simulink model "Torque_controller"  (R2023b)
settings: Solver=VariableStepAuto  StartTime=0.0  StopTime=50  RelTol=1e-3
values from neighbouring files (symbols this model uses):
  b = 0.016    [torque.m]
  Im = 0.059    [torque.m]
  k = kt    (= 1.45433391507)    [torque.m]
  L = 0.01    [torque.m]
  R = 2.0    (= 2)    [torque.m]
libraries: cstblocks x1
settings Model: Creator=giova  LastModifiedBy=david

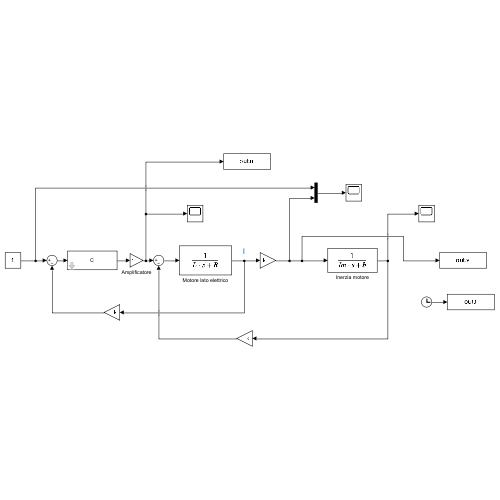
[thumbnail: Simulink's stored preview of the top-level diagram]
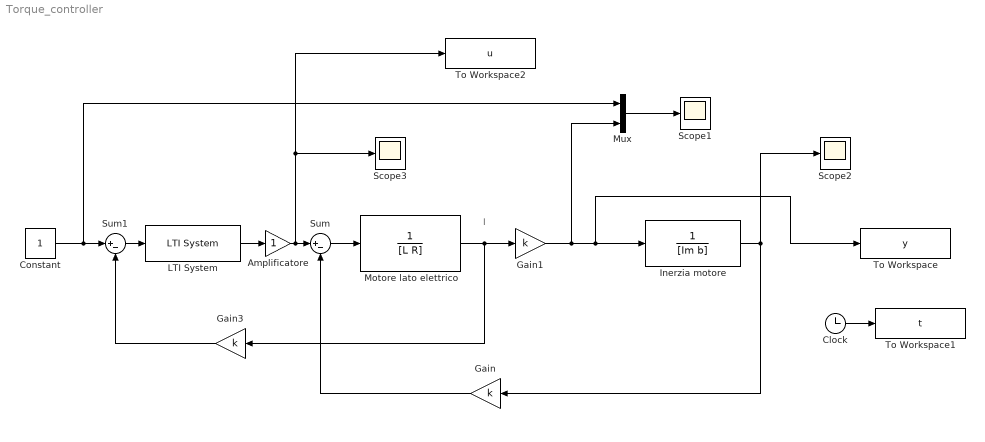
== system Torque_controller ==
  note: I
  Amplificatore : Gain
  Clock : Clock
  Constant : Constant
  Gain : Gain  Gain=k
  Gain1 : Gain  Gain=k
  Gain3 : Gain  Gain=k
  Inerzia motore : TransferFcn  Denominator=[Im b]
  LTI System : cstblocks/LTI System  sys=C  IC=[]  PadeOrder=0
  Motore lato elettrico : TransferFcn  Denominator=[L R]
  Mux : Mux  Inputs=2
  Scope1 : Scope
  Scope2 : Scope
  Scope3 : Scope
  Sum : Sum  Inputs=|+-
  Sum1 : Sum  Inputs=|+-
  To Workspace : ToWorkspace  VariableName=y  SampleTime=-1
  To Workspace1 : ToWorkspace  VariableName=t  SampleTime=-1
  To Workspace2 : ToWorkspace  VariableName=u  SampleTime=-1
  wires:
  Clock/1 -> To Workspace1/1
  Gain1/1 -> Mux/2, To Workspace/1, Inerzia motore/1
  Motore lato elettrico/1 -> Gain1/1, Gain3/1
  Sum/1 -> Motore lato elettrico/1
  Inerzia motore/1 -> Gain/1, Scope2/1
  Gain/1 -> Sum/2
  Constant/1 -> Mux/1, Sum1/1
  Mux/1 -> Scope1/1
  Sum1/1 -> LTI System/1
  LTI System/1 -> Amplificatore/1
  Amplificatore/1 -> To Workspace2/1, Scope3/1, Sum/1
  Gain3/1 -> Sum1/2
